simulink model "nonlinearAirframe"  (R2024b)
settings: Solver=ode3  StartTime=0  StopTime=10.0  FixedStep=Ts  RelTol=1e-3  EnableMultiTasking=on
undefined symbols (not defined in the file): Earth, initPosLLA, Vehicle, WGS84, zylo
libraries: actuatorsLibrary x3, shared6dof x1, aerolibasang x1, aerolibtransform2 x1
settings Model: Creator=The MathWorks, Inc.  LastModifiedBy=isaac
settings SolverCC: AlgebraicLoopSolver=TrustRegion  AutoInsertRateTranBlk=on
settings DataIOCC: SaveFormat=Array  SaveOutput=off  SignalLogging=off  DSMLogging=off  SaveTime=off  ReturnWorkspaceOutputs=off
settings OptimizationCC: BlockReduction=off  DefaultParameterBehavior=Inlined  BufferReuse=off  LifeSpan=inf
settings DebuggingCC: AlgebraicLoopMsg=none  UnderspecifiedInitializationDetection=Classic  MergeDetectMultiDrivingBlocksExec=none  AllowSymbolicDim=off  SFUnexpectedBacktrackingDiag=warning  SFNoUnconditionalDefaultTransitionDiag=warning  SFExecutionAtInitializationDiag=none  ArithmeticOperatorsInVariantConditions=warning
settings HardwareCC: ProdBitPerPointer=32  ProdBitPerSizeT=32  ProdBitPerPtrDiffT=32  ProdLargestAtomicFloat=None  ProdIntDivRoundTo=Undefined  ProdEndianess=Unspecified  ProdWordSize=32  ProdHWDeviceType=32-bit Generic
settings ModelReferenceCC: EnableRefExpFcnMdlSchedulingChecks=on  PropagateSignalLabelsOutOfModel=off
settings SFSimCC: SimUseLocalCustomCode=off
settings RTWCC: RTWUseLocalCustomCode=off  GPUComputeCapability=3.5
settings CodeAppCC: StateflowObjectComments=on
settings GRTTargetCC: TargetLangStandard=C89/C90 (ANSI)
settings ConfigComp: CovMetricSettings=dw  CovSaveCumulativeToWorkspaceVar=on  CovSaveSingleToWorkspaceVar=on  CovExternalEMLEnable=off  CovSFcnEnable=off

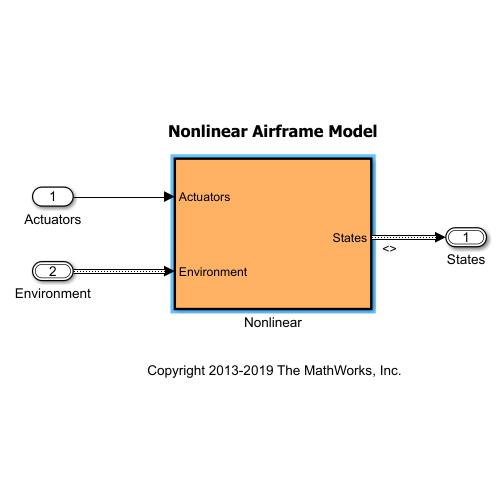
[thumbnail: Simulink's stored preview of the top-level diagram]
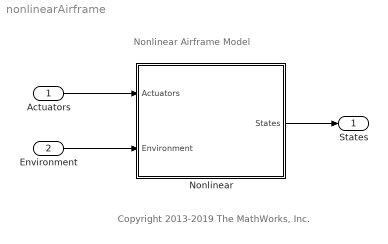
== system nonlinearAirframe ==
  note: Copyright 2013-2019 The MathWorks, Inc.
  note: Nonlinear Airframe Model
  Actuators : Inport
  Environment : Inport  Port=2  OutDataTypeStr=Bus: EnvironmentBus  BusOutputAsStruct=on
  Nonlinear : Subsystem  TreatAsAtomicUnit=on
      mask init:
      | vehicleNonlinearVars;
  States : Outport  OutDataTypeStr=Bus: StatesBus  VectorParamsAs1DForOutWhenUnconnected=off  BusOutputAsStruct=on
  wires:
  Actuators/1 -> Nonlinear/1(Actuators)
  Environment/1 -> Nonlinear/2(Environment)
  Nonlinear/1(States) -> States/1

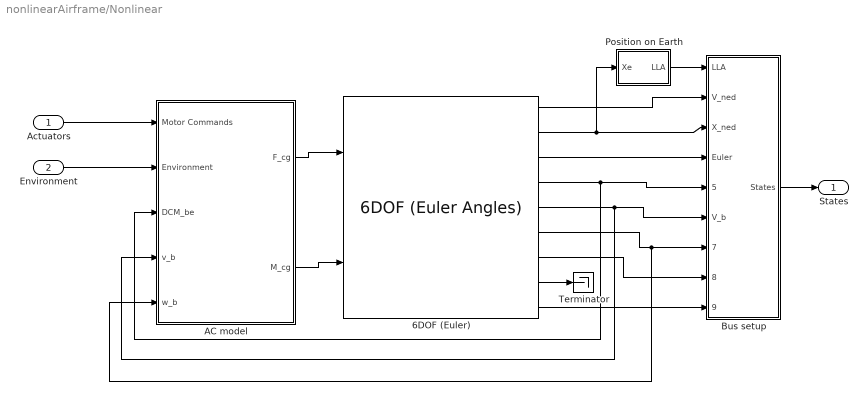
== system nonlinearAirframe/Nonlinear ==
  Actuators : Inport
  Environment : Inport  Port=2
  6DOF (Euler) : shared6dof/6DOF (Euler Angles)  units=Metric (MKS)  mtype=Fixed  rep=Euler Angles  xme_0=initPosNED  Vm_0=initVb  eul_0=initEuler  pm_0=initAngRates  mass_0=mass  mass_e=0.5  mass_f=2.0  inertia=inertia  inertia_e=eye(3)  inertia_f=2*eye(3)  k_quat=Vehicle.Nonlinear.Nonlinear.SixDOF.quatGain  vre_flag=on  abi_flag=on  aMode=aMode  xme_statename=''  Vm_statename=''  eul_statename=''  quat_statename=''  pm_statename=''  mass_statename=''
  AC model : Subsystem
  Bus setup : Subsystem
  Position on Earth : Subsystem  Priority=1  TreatAsAtomicUnit=on
  Terminator : Terminator
  States : Outport  VectorParamsAs1DForOutWhenUnconnected=off
  wires:
  Actuators/1 -> AC model/1(Motor Commands)
  Environment/1 -> AC model/2(Environment)
  AC model/1(F_cg) -> 6DOF (Euler)/1
  AC model/2(M_cg) -> 6DOF (Euler)/2
  6DOF (Euler)/1 -> Bus setup/2(V_ned)
  6DOF (Euler)/2 -> Position on Earth/1(Xe), Bus setup/3(X_ned)
  6DOF (Euler)/3 -> Bus setup/4(Euler)
  6DOF (Euler)/4 -> AC model/3(DCM_be), Bus setup/5(DCM_be)
  6DOF (Euler)/5 -> AC model/4(v_b), Bus setup/6(V_b)
  6DOF (Euler)/6 -> AC model/5(w_b), Bus setup/7(Omega_b)
  6DOF (Euler)/7 -> Bus setup/8(dOmega_b)
  Position on Earth/1(LLA) -> Bus setup/1(LLA)
  Bus setup/1(States) -> States/1
  6DOF (Euler)/9 -> Bus setup/9(Accel_b)
  6DOF (Euler)/8 -> Terminator/1

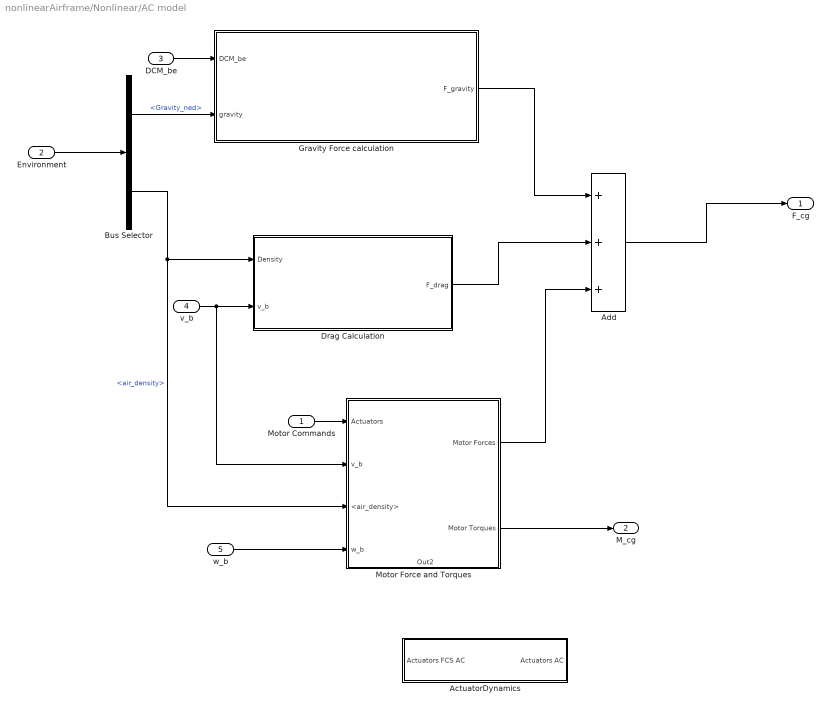
== system nonlinearAirframe/Nonlinear/AC model ==
  Motor Commands : Inport
  Environment : Inport  Port=2
  DCM_be : Inport  Port=3
  v_b : Inport  Port=4
  w_b : Inport  Port=5
  ActuatorDynamics : Subsystem  Variant=on
  Add : Sum  Inputs=+++
  Bus Selector : BusSelector  OutputSignals=Gravity_ned,AtmosphereBus.air_density
  Drag Calculation : Subsystem
  Gravity Force calculation : Subsystem
  Motor Force and Torques : Subsystem
      settings: PortSchema="{\"entries\":[{\"content\":{\"sides\":[{\"content\":{\"connectorIds\":[\"In1\",\"In2\",\"In3\",\"In4\"]},\"type\":\"ConnectorPlacement.EquallySpacedRectSide\",\"uuid\":\"39d241ed-5105-479b-b2d4-25b5fcc7d112\"},{\"content\":{\"connectorIds\":[\"Out1\",\"Out2\"],\"side\":\"RIGHT\"},\"type\":\"ConnectorPlacement.EquallySpacedRectSide\",\"uuid\":\"3b54dc2a-7bdd-4451-8de0-2896ca18812b\"},{\"content\":{\"side\":\"TOP\"},\"type\":\"ConnectorPlacement.EquallySpacedRectSide\",\"uuid\":\"596166b3-3aaf-4093-9878-566715d230fd\"},{\"content\":{\"connectorIds\":[\"Out3\"],\"side\":\"BOTTOM\"},\"type\":\"ConnectorPlacement.EquallySpacedRectSide\",\"uuid\":\"35f53c90-72bc-4547-98fd-a785a69c1239\"}]},\"type\":\"ConnectorPlacement.EquallySpacedConnector\",\"uuid\":\"8a8f87bb-adbe-431f-b05d-4bb99aa16baa\"}],\"packageUris\":[\"http://schema.mathworks.com/mf0/Connector/R2020b\"],\"version\":\"1.0\"}"
  F_cg : Outport  VectorParamsAs1DForOutWhenUnconnected=off
  M_cg : Outport  Port=2  VectorParamsAs1DForOutWhenUnconnected=off
  wires:
  Environment/1 -> Bus Selector/1
  Add/1 -> F_cg/1
  Motor Commands/1 -> Motor Force and Torques/1(Actuators)
  Bus Selector/1 -> Gravity Force calculation/2(gravity)  "<Gravity_ned>"
  DCM_be/1 -> Gravity Force calculation/1(DCM_be)
  Bus Selector/2 -> Motor Force and Torques/3(<air_density>), Drag Calculation/1(Density)  "<air_density>"
  v_b/1 -> Motor Force and Torques/2(v_b), Drag Calculation/2(v_b)
  w_b/1 -> Motor Force and Torques/4(w_b)
  Motor Force and Torques/2(Motor Torques) -> M_cg/1
  Motor Force and Torques/1(Motor Forces) -> Add/3
  Drag Calculation/1(F_drag) -> Add/2
  Gravity Force calculation/1(F_gravity) -> Add/1

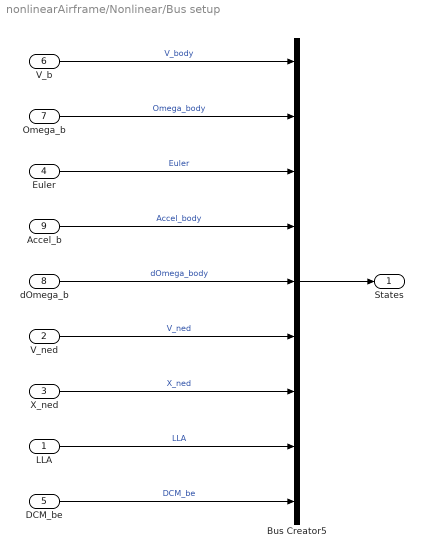
== system nonlinearAirframe/Nonlinear/Bus setup ==
  LLA : Inport  PortDimensions=3
  V_ned : Inport  Port=2  PortDimensions=3
  X_ned : Inport  Port=3  PortDimensions=3
  Euler : Inport  Port=4  PortDimensions=3
  DCM_be : Inport  Port=5  PortDimensions=[3 3]
  V_b : Inport  Port=6  PortDimensions=3
  Omega_b : Inport  Port=7  PortDimensions=3
  dOmega_b : Inport  Port=8  PortDimensions=3
  Accel_b : Inport  Port=9  PortDimensions=3
  Bus Creator5 : BusCreator  Inputs=9  OutDataTypeStr=Bus: StatesBus  NonVirtualBus=on
  States : Outport  VectorParamsAs1DForOutWhenUnconnected=off
  wires:
  Bus Creator5/1 -> States/1
  V_b/1 -> Bus Creator5/1  "V_body"
  Omega_b/1 -> Bus Creator5/2  "Omega_body"
  Euler/1 -> Bus Creator5/3  "Euler"
  X_ned/1 -> Bus Creator5/7  "X_ned"
  Accel_b/1 -> Bus Creator5/4  "Accel_body"
  LLA/1 -> Bus Creator5/8  "LLA"
  dOmega_b/1 -> Bus Creator5/5  "dOmega_body"
  DCM_be/1 -> Bus Creator5/9  "DCM_be"
  V_ned/1 -> Bus Creator5/6  "V_ned"

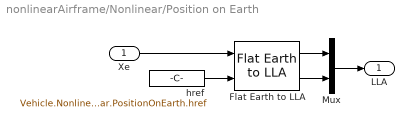
== system nonlinearAirframe/Nonlinear/Position on Earth ==
  Xe : Inport
  Flat Earth to LLA : aerolibtransform2/Flat Earth to LLA  units=Metric (MKS)  ptype=Earth (WGS84)  F=1/298.257223563  R=6378137  refPosPort=off  LL0=initPosLLA(1:2)  psi=Vehicle.Nonlinear.Nonlinear.PositionOnEarth.FlatEarthToLLA.xAxis
  Mux : Mux  Inputs=2
  href : Constant  Value=Vehicle.Nonlinear.Nonlinear.PositionOnEarth.href
  LLA : Outport  VectorParamsAs1DForOutWhenUnconnected=off
  wires:
  Mux/1 -> LLA/1
  Xe/1 -> Flat Earth to LLA/1
  Flat Earth to LLA/1 -> Mux/1
  Flat Earth to LLA/2 -> Mux/2
  href/1 -> Flat Earth to LLA/2

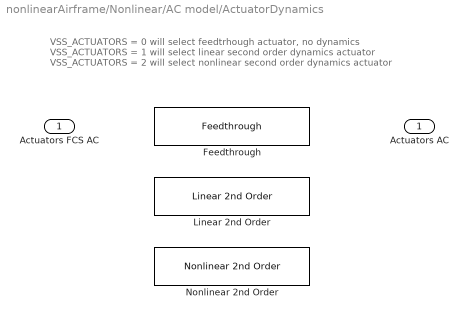
== system nonlinearAirframe/Nonlinear/AC model/ActuatorDynamics ==
  note: VSS_ACTUATORS = 0 will select feedtrhough actuator, no dynamics
      | VSS_ACTUATORS = 1 will select linear second order dynamics actuator
      | VSS_ACTUATORS = 2 will select nonlinear second order dynamics actuator
  Actuators FCS AC : Inport
  Feedthrough : actuatorsLibrary/Feedthrough  SystemSampleTime=-1  VariantControl=VSS_ACTUATORS_FEEDTHROUGH  VariantActivationTime=update diagram  AllowFlexibleInterface=on  Latency=0  AutoFrameSizeCalculation=off
  Linear 2nd Order : actuatorsLibrary/Linear 2nd Order  SystemSampleTime=-1  VariantControl=VSS_ACTUATORS_LINEAR  VariantActivationTime=update diagram  AllowFlexibleInterface=on  Latency=0  AutoFrameSizeCalculation=off
  Nonlinear 2nd Order : actuatorsLibrary/Nonlinear 2nd Order  SystemSampleTime=-1  VariantControl=VSS_ACTUATORS_NONLINEAR  VariantActivationTime=update diagram  AllowFlexibleInterface=on  Latency=0  AutoFrameSizeCalculation=off
  Actuators AC : Outport  VectorParamsAs1DForOutWhenUnconnected=off

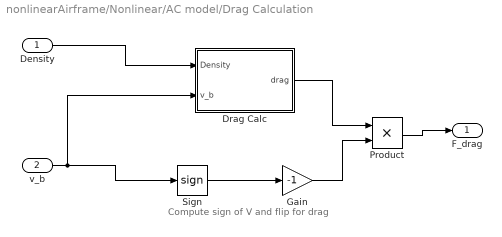
== system nonlinearAirframe/Nonlinear/AC model/Drag Calculation ==
  note: Compute sign of V and flip for drag
  Density : Inport
  v_b : Inport  Port=2
  Drag Calc : Subsystem
  Gain : Gain  Gain=-1
  Product : Product
  Sign : Signum
  F_drag : Outport
  wires:
  v_b/1 -> Drag Calc/2(v_b), Sign/1
  Sign/1 -> Gain/1
  Gain/1 -> Product/2
  Density/1 -> Drag Calc/1(Density)
  Drag Calc/1(drag) -> Product/1
  Product/1 -> F_drag/1

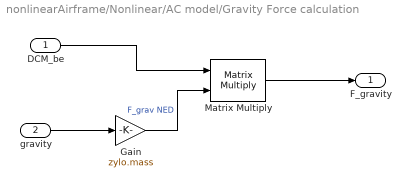
== system nonlinearAirframe/Nonlinear/AC model/Gravity Force calculation ==
  DCM_be : Inport
  gravity : Inport  Port=2
  Gain : Gain  Gain=zylo.mass
  Matrix Multiply : Product  Multiplication=Matrix(*)
  F_gravity : Outport
  wires:
  gravity/1 -> Gain/1
  DCM_be/1 -> Matrix Multiply/1
  Gain/1 -> Matrix Multiply/2  "F_grav NED"
  Matrix Multiply/1 -> F_gravity/1

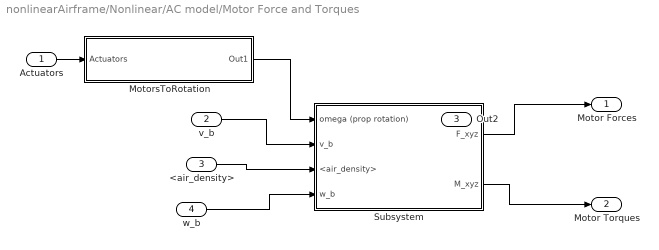
== system nonlinearAirframe/Nonlinear/AC model/Motor Force and Torques ==
  Actuators : Inport
  v_b : Inport  Port=2
  <air_density> : Inport  Port=3
  w_b : Inport  Port=4
  MotorsToRotation : Subsystem
  Subsystem : Subsystem
  Motor Forces : Outport
  Motor Torques : Outport  Port=2
  Out2 : Outport  Port=3
  wires:
  Actuators/1 -> MotorsToRotation/1(Actuators)
  <air_density>/1 -> Subsystem/3(<air_density>)
  v_b/1 -> Subsystem/2(v_b)
  MotorsToRotation/1(Out1) -> Subsystem/1(omega (prop rotation))
  w_b/1 -> Subsystem/4(w_b)
  Subsystem/2(M_xyz) -> Motor Torques/1
  Subsystem/1(F_xyz) -> Motor Forces/1

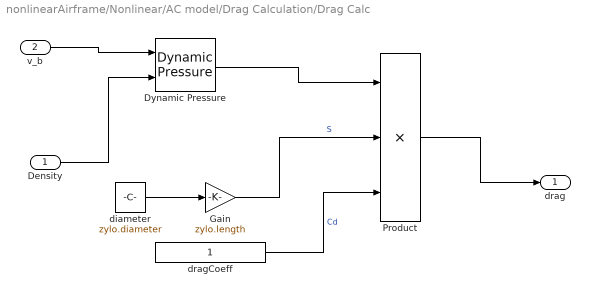
== system nonlinearAirframe/Nonlinear/AC model/Drag Calculation/Drag Calc ==
  Density : Inport
  v_b : Inport  Port=2
  Dynamic Pressure : aerolibasang/Dynamic Pressure
  Gain : Gain  Gain=zylo.length
  Product : Product  Inputs=3
  diameter : Constant  Value=zylo.diameter
  dragCoeff : Constant
  drag : Outport
  wires:
  Density/1 -> Dynamic Pressure/2
  v_b/1 -> Dynamic Pressure/1
  Dynamic Pressure/1 -> Product/1
  dragCoeff/1 -> Product/3  "Cd"
  Gain/1 -> Product/2  "S"
  diameter/1 -> Gain/1
  Product/1 -> drag/1

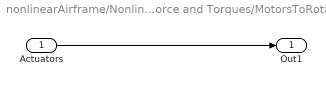
== system nonlinearAirframe/Nonlinear/AC model/Motor Force and Torques/MotorsToRotation ==
  Actuators : Inport
  Out1 : Outport
  wires:
  Actuators/1 -> Out1/1

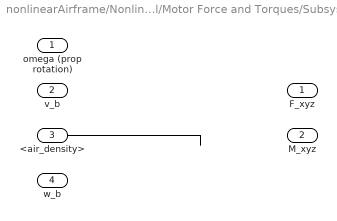
== system nonlinearAirframe/Nonlinear/AC model/Motor Force and Torques/Subsystem ==
  omega (prop rotation) : Inport
  v_b : Inport  Port=2
  <air_density> : Inport  Port=3
  w_b : Inport  Port=4
  F_xyz : Outport
  M_xyz : Outport  Port=2
  wires:
  <air_density>/1 -> ?
